simulink model "Engine"  (R2025a)
settings: Solver=VariableStepAuto  StartTime=0.0  StopTime=15  RelTol=1e-3
undefined symbols (not defined in the file): Cm, Cw, Jdv, Lj, Lov, Rj
libraries: SignalEditorBlockLib x1
settings Model: Creator=Reymond  LastModifiedBy=Reymond

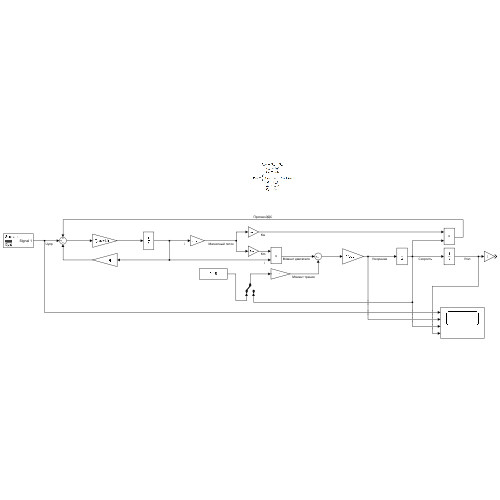
[thumbnail: Simulink's stored preview of the top-level diagram]
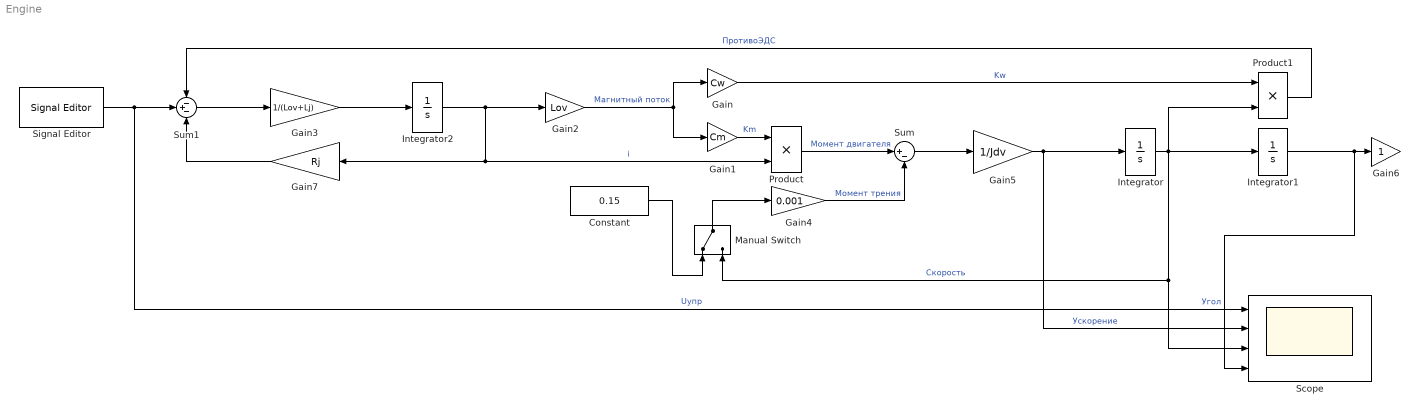
== system Engine ==
  Constant : Constant  Value=0.15
  Gain : Gain  Gain=Cw
  Gain1 : Gain  Gain=Cm
  Gain2 : Gain  Gain=Lov
  Gain3 : Gain  Gain=1/(Lov+Lj)
  Gain4 : Gain  Gain=0.001
  Gain5 : Gain  Gain=1/Jdv
  Gain6 : Gain
  Gain7 : Gain  Gain=Rj
  Integrator : Integrator
  Integrator1 : Integrator
  Integrator2 : Integrator
  Manual Switch : ManualSwitch
  Product : Product
  Product1 : Product
  Scope : Scope  NumInputPorts=4
      settings: ActiveDisplayYMinimum=-0.62368454116953476  ActiveDisplayYMaximum=5.6131608705258138
  Signal Editor : SignalEditorBlockLib/Signal Editor  FileName=signal.mat  ActiveScenario=Scenario  ActiveSignal=Signal 1  IsBus=off  OutputBusObjectStr=Bus: BusObject  SampleTime=0  ZeroCross=off  OutputAfterFinalValue=Setting to zero  Unit=inherit  PreserveSignalName=on  ApplySigPropsToAllScenarios=on  ApplySigPropsToAllSignals=off  SignalPropertySource=Dialog parameters
  Sum : Sum  Inputs=|+-
  Sum1 : Sum  Inputs=-+-
  wires:
  Gain2/1 -> Gain/1, Gain1/1  "Магнитный поток"
  Integrator2/1 -> Gain7/1, Product/2, Gain2/1  "i"
  Gain1/1 -> Product/1  "Km"
  Product/1 -> Sum/1  "Момент двигателя"
  Gain4/1 -> Sum/2  "Момент трения"
  Sum/1 -> Gain5/1
  Gain5/1 -> Scope/2, Integrator/1  "Ускорение"
  Integrator/1 -> Manual Switch/2, Scope/3, Product1/2, Integrator1/1  "Скорость"
  Integrator1/1 -> Scope/4, Gain6/1  "Угол"
  Gain/1 -> Product1/1  "Kw"
  Signal Editor/1 -> Scope/1, Sum1/2  "Uупр"
  Sum1/1 -> Gain3/1
  Gain3/1 -> Integrator2/1
  Gain7/1 -> Sum1/3
  Product1/1 -> Sum1/1  "ПротивоЭДС"
  Constant/1 -> Manual Switch/1
  Manual Switch/1 -> Gain4/1
